simulink model "Factorial"  (R2021a)
settings: Solver=VariableStepAuto  StartTime=0.0  StopTime=10.0  RelTol=1e-3
settings Model: Creator=AL_hamd  LastModifiedBy=AL_hamd

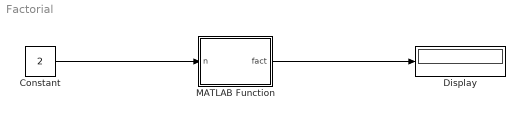
== system Factorial ==
  Constant : Constant  Value=2
  Display : Display
  MATLAB Function : MATLAB Function  TreatAsAtomicUnit=on
  wires:
  MATLAB Function/1(fact) -> Display/1
  Constant/1 -> MATLAB Function/1(n)

== matlab function Factorial/MATLAB Function ==
  data: n input; fact output
function fact = fcn(n)
fact =1;
for i=1:n
    fact = fact*i;
end
end
